simulink model "LKA_and_ELK_State_Machine"  (R2018b)
settings: Solver=VariableStepAuto  StartTime=0.0  StopTime=10.0  RelTol=1e-3
settings Model: Creator=hejr  LastModifiedBy=xiaoyang

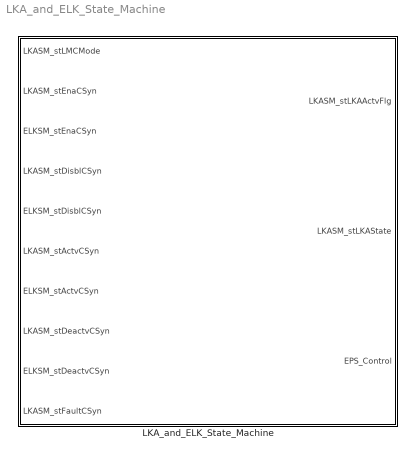
== system LKA_and_ELK_State_Machine ==
  LKA_and_ELK_State_Machine : Stateflow chart  Description=|  TreatAsAtomicUnit=on
      | Block Name: LKA State Machine
      | Ab.: LKASM
      | No.: 1.1.3.0
      | Rev: 0.0.1
      | Update Date: 19-3-26
      settings: RTWSystemCode=Nonreusable function

== stateflow chart LKA_and_ELK_State_Machine/LKA_and_ELK_State_Machine ==
  state SysOn
    state LKASelected
      en:
      LKASM_stLKAState = uint8(2);
    state Normal
      state LKA_Enable
        en:
        EPS_Control = uint8(1);
        ex:
        EPS_Control = uint8(0);
        state LKAEnable
          en:
          LKASM_stLKAState = uint8(3);
          EPS_Control = uint8(1)
        state LKALeftActive
          en:
          LKASM_stLKAState = uint8(4);
          LKASM_stLKAActvFlg = LKASM_stActvCSyn;
          ex:
          LKASM_stLKAActvFlg = uint8(0);
        state LKARightActive
          en:
          LKASM_stLKAState = uint8(5);
          LKASM_stLKAActvFlg = LKASM_stActvCSyn;
          ex:
          LKASM_stLKAActvFlg = uint8(0);
        (default) -> LKAEnable
        LKAEnable -> LKALeftActive [order 2] : [LKASM_stActvCSyn == 1 & LKASM_stDeactvCSyn ==0 ]
        LKAEnable -> LKARightActive [order 1] : [LKASM_stActvCSyn == 2 & LKASM_stDeactvCSyn ==0 ]
        LKALeftActive -> LKAEnable [order 1] : [LKASM_stDeactvCSyn ==1 ]
        LKARightActive -> LKAEnable [order 1] : [LKASM_stDeactvCSyn == 1]
        LKALeftActive -> LKARightActive [order 2] : [LKASM_stActvCSyn == 2 & LKASM_stDeactvCSyn ==0]
        LKARightActive -> LKALeftActive [order 2] : [LKASM_stActvCSyn == 1 & LKASM_stDeactvCSyn ==0]
      state ELK_Enable
        en:
        EPS_Control = uint8(2);
        ex:
        EPS_Control = uint8(0);
        state ELKEnable
          en:
          LKASM_stLKAState = uint8(3);
        state ELKLeftActive
          en:
          LKASM_stLKAState = uint8(4);
          LKASM_stLKAActvFlg = ELKSM_stActvCSyn;
          ex:
          LKASM_stLKAActvFlg = uint8(0);
        state ELKRightActive
          en:
          LKASM_stLKAState = uint8(5);
          LKASM_stLKAActvFlg = ELKSM_stActvCSyn;
          ex:
          LKASM_stLKAActvFlg = uint8(0);
        (default) -> ELKEnable
        ELKEnable -> ELKLeftActive [order 2] : [ELKSM_stActvCSyn < 15 & ELKSM_stDeactvCSyn ==0 ]
        ELKEnable -> ELKRightActive [order 1] : [ELKSM_stActvCSyn > 15 & ELKSM_stDeactvCSyn ==0 ]
        ELKLeftActive -> ELKEnable [order 2] : [ELKSM_stDeactvCSyn == 1]
        ELKRightActive -> ELKEnable [order 2] : [ELKSM_stDeactvCSyn == 1]
        ELKLeftActive -> ELKRightActive [order 1] : [ELKSM_stActvCSyn > 15 & ELKSM_stDeactvCSyn ==0]
        ELKRightActive -> ELKLeftActive [order 1] : [ELKSM_stActvCSyn < 15 & ELKSM_stDeactvCSyn ==0]
      (junction 121) -> LKA_Enable [order 2] : [(LKASM_stEnaCSyn == 1 & LKASM_stDisblCSyn ==0) ]
      (junction 121) -> ELK_Enable [order 1] : [(ELKSM_stEnaCSyn == 1 & ELKSM_stDisblCSyn ==0)]
      ELK_Enable -> (junction 121) : [ELKSM_stDisblCSyn ==1]
      LKA_Enable -> (junction 121) : [LKASM_stDisblCSyn ==1]
    (default) -> LKASelected
    LKASelected -> LKA_Enable [order 2] : [(LKASM_stEnaCSyn == 1 & LKASM_stDisblCSyn ==0) ]
    (junction 121) -> LKASelected [order 3]
    Normal -> LKASelected : [(LKASM_stDisblCSyn ==1 & ELKSM_stDisblCSyn ==1)]
    LKASelected -> ELK_Enable [order 1] : [(ELKSM_stEnaCSyn == 1 & ELKSM_stDisblCSyn ==0)]
  state SysOff
    state Unselected
      en:
      LKASM_stLKAState = uint8(1);
    state Unavailable
      en:
      LKASM_stLKAState = uint8(0);
    (default) -> Unavailable
    Unavailable -> Unselected : [LKASM_stLMCMode == 0 | LKASM_stLMCMode == 1]
  state LKAFault
    en:
    LKASM_stLKAState = uint8(6);
  (default) -> SysOff
  SysOff -> SysOn [order 2] : [LKASM_stLMCMode == 2|LKASM_stLMCMode == 3]
  SysOn -> Unselected [order 2] : [LKASM_stLMCMode ~= 2&LKASM_stLMCMode ~= 3]
  LKAFault -> Unselected [order 2] : [(LKASM_stLMCMode == 0 | LKASM_stLMCMode == 1) & LKASM_stFaultCSyn == 0]
  SysOff -> LKAFault [order 1] : [(LKASM_stLMCMode == 2|LKASM_stLMCMode == 3) & LKASM_stFaultCSyn == 1 ]
  SysOn -> LKAFault [order 1] : [LKASM_stFaultCSyn == 1 ]
  LKAFault -> SysOn [order 1] : [LKASM_stFaultCSyn == 0 & (LKASM_stLMCMode == 2|LKASM_stLMCMode == 3)]
  data: LKASM_stLKAActvFlg output uint8 [0..7]; LKASM_stLKAState output uint8 [0..7]; LKASM_stLMCMode input uint8 [0..5]; LKASM_stEnaCSyn input boolean [0..1]; ELKSM_stEnaCSyn input boolean; LKASM_stDisblCSyn input boolean [0..1]; ELKSM_stDisblCSyn input boolean; LKASM_stActvCSyn input uint8 [0..3]; ELKSM_stActvCSyn input uint8; LKASM_stDeactvCSyn input boolean [0..1]; ELKSM_stDeactvCSyn input boolean; LKASM_stFaultCSyn input boolean [0..1]; EPS_Control output uint8
  data LKASM_stLKAActvFlg settings: description=|
      | 0 -- Deactive
      | 1 -- Left Active
      | 2 -- Right Active
  data LKASM_stLKAState settings: description=|
      | 0 -- Unavailable
      | 1 -- Unselected
      | 2 -- Selected
      | 3 -- Enabled
      | 4 -- Left Active
      | 5 -- Right Active
      | 6 -- Fault
      | 7 -- Reserved
  data LKASM_stLMCMode settings: description=|
      | 0 -- Unselected
      | 1 -- LDWMode
      | 2 -- LKAMode
      | 3 -- TJAMode
      | 4 -- HWAMode
      | 5 -- Reserved
  data LKASM_stEnaCSyn settings: description=|
      | 0 -- No Enable
      | 1 -- LDW Enable
      | 2 -- LKA Enable
      | 3 -- Reserved
  data LKASM_stDisblCSyn settings: description=|
      | 0 -- No Disable
      | 1 -- LDW Disable
      | 2 -- LKA Disable
      | 3 -- Reserved
  data LKASM_stActvCSyn settings: description=|
      | 0 -- No Active
      | 1 -- LDW Left Active
      | 2 -- LDW Right Active
      | 3 -- LKA Left Active
      | 4 -- LKA Right Active
      | 5 -- Reserved
  data LKASM_stDeactvCSyn settings: description=|
      | 0 -- No Deactive
      | 1 -- LDW Deactive
      | 2 -- LKA Deactive
      | 3 -- Reserved
  data LKASM_stFaultCSyn settings: description=|
      | 0 -- No Fault
      | 1 -- LDW Fault
      | 2 -- LKA Fault
      | 3 -- Reserved
